simulink model "CLIK_inv_jacob_2order"  (R2021a)
settings: Solver=VariableStepAuto  StartTime=0.0  StopTime=50  RelTol=1e-3
values from neighbouring files (symbols this model uses):
  KD = kdi*eye(4)    [traiettoria.m]
  KP = kpi*eye(4)    [traiettoria.m]
  q0 = scara.ikine(T0, 'mask', [1 1 1 1 0 0])    [pseudo_traiettoria.m]    (also in traiettoria.m)
  Tc = 0.001    [pseudo_traiettoria.m]    (also in traiettoria.m)
undefined symbols (not defined in the file or in its folder): DiscIntNeverNeededParam
settings Model: Creator=Ciro  LastModifiedBy=Ciro

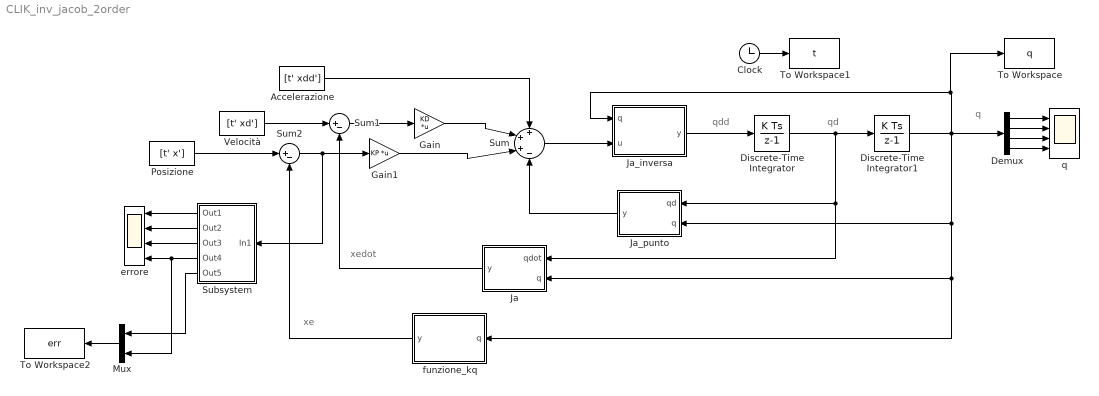
== system CLIK_inv_jacob_2order ==
  note: qd
  note: xedot
  note: qdd
  note: q
  note: xe
  Accelerazione : FromWorkspace  VariableName=[t' xdd']  SampleTime=Tc  OutputAfterFinalValue=Holding final value
  Clock : Clock
  Demux : Demux
  Discrete-Time Integrator : DiscreteIntegrator  InitialCondition=[0; 0; 0; 0]  SampleTime=Tc  ICPrevOutput=DiscIntNeverNeededParam  ICPrevScaledInput=DiscIntNeverNeededParam
  Discrete-Time Integrator1 : DiscreteIntegrator  InitialCondition=q0  SampleTime=Tc  ICPrevOutput=DiscIntNeverNeededParam  ICPrevScaledInput=DiscIntNeverNeededParam
  Gain : Gain  Gain=KD  Multiplication=Matrix(K*u)
  Gain1 : Gain  Gain=KP  Multiplication=Matrix(K*u)
  Ja : MATLAB Function  TreatAsAtomicUnit=on
  Ja_inversa : MATLAB Function  TreatAsAtomicUnit=on
  Ja_punto : MATLAB Function  TreatAsAtomicUnit=on
  Mux : Mux  Inputs=2
  Posizione : FromWorkspace  VariableName=[t' x']  SampleTime=Tc  OutputAfterFinalValue=Holding final value
  Subsystem : Subsystem
  Sum : Sum  Inputs=+++-
  Sum1 : Sum  Inputs=|+-
  Sum2 : Sum  Inputs=|+-
  To Workspace : ToWorkspace  VariableName=q  SampleTime=-1
      settings: Save2DSignal=2-D array (concatenate along first dimension)
  To Workspace1 : ToWorkspace  VariableName=t  SampleTime=-1
      settings: Save2DSignal=2-D array (concatenate along first dimension)
  To Workspace2 : ToWorkspace  VariableName=err  SampleTime=-1
      settings: Save2DSignal=2-D array (concatenate along first dimension)
  Velocità : FromWorkspace  VariableName=[t' xd']  SampleTime=Tc  OutputAfterFinalValue=Holding final value
  errore : Scope  NumInputPorts=4
  funzione_kq : MATLAB Function  TreatAsAtomicUnit=on
  q : Scope  NumInputPorts=4
  wires:
  Discrete-Time Integrator1/1 -> To Workspace/1, Ja_inversa/1(q), Demux/1, funzione_kq/1(q), Ja/2(q), Ja_punto/2(q)
  Discrete-Time Integrator/1 -> Ja/1(qdot), Ja_punto/1(qd), Discrete-Time Integrator1/1
  Ja/1(y) -> Sum1/2
  Ja_punto/1(y) -> Sum/4
  funzione_kq/1(y) -> Sum2/2
  Gain1/1 -> Sum/3
  Ja_inversa/1(y) -> Discrete-Time Integrator/1
  Sum/1 -> Ja_inversa/2(u)
  Gain/1 -> Sum/2
  Accelerazione/1 -> Sum/1
  Velocità/1 -> Sum1/1
  Demux/1 -> q/1
  Demux/2 -> q/2
  Demux/3 -> q/3
  Demux/4 -> q/4
  Sum2/1 -> Subsystem/1(In1), Gain1/1
  Sum1/1 -> Gain/1
  Posizione/1 -> Sum2/1
  Clock/1 -> To Workspace1/1
  Subsystem/3(Out3) -> errore/3
  Subsystem/2(Out2) -> errore/2
  Subsystem/1(Out1) -> errore/1
  Subsystem/4(Out4) -> Mux/2, errore/4
  Mux/1 -> To Workspace2/1
  Subsystem/5(Out5) -> Mux/1

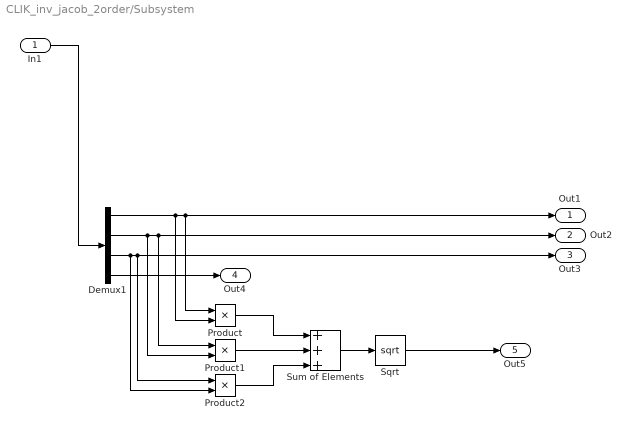
== system CLIK_inv_jacob_2order/Subsystem ==
  In1 : Inport
  Demux1 : Demux
  Product : Product
  Product1 : Product
  Product2 : Product
  Sqrt : Sqrt  SaturateOnIntegerOverflow=on
  Sum of Elements : Sum  Inputs=+++
  Out1 : Outport
  Out2 : Outport  Port=2
  Out3 : Outport  Port=3
  Out4 : Outport  Port=4
  Out5 : Outport  Port=5
  wires:
  Demux1/3 -> Product2/2, Out3/1, Product2/1
  Demux1/2 -> Product1/2, Out2/1, Product1/1
  Product/1 -> Sum of Elements/1
  Sum of Elements/1 -> Sqrt/1
  Product1/1 -> Sum of Elements/2
  Demux1/4 -> Out4/1
  Demux1/1 -> Product/2, Out1/1, Product/1
  Product2/1 -> Sum of Elements/3
  Sqrt/1 -> Out5/1
  In1/1 -> Demux1/1

== matlab function CLIK_inv_jacob_2order/Ja_inversa ==
  data: q input; u input; y output
function y = fcn(q, u)
J = [ -0.5*(sin(q(1))+sin(q(1)+q(2))) -0.5*sin(q(1)+q(2))  0  0;
       0.5*(cos(q(1))+cos(q(1)+q(2)))  0.5*cos(q(1)+q(2))  0  0;
       0                               0                  -1  0;
       1                               1                   0 -1];
y = inv(J)*u;

== matlab function CLIK_inv_jacob_2order/Ja ==
  data: qdot input; q input; y output
function y = fcn(qdot,q)
J = [ -0.5*(sin(q(1))+sin(q(1)+q(2))) -0.5*sin(q(1)+q(2))  0  0;
       0.5*(cos(q(1))+cos(q(1)+q(2)))  0.5*cos(q(1)+q(2))  0  0;
       0                               0                  -1  0;
       1                               1                   0 -1];
y = J*qdot;

== matlab function CLIK_inv_jacob_2order/Ja_punto ==
  data: qd input; q input; y output
function y = fcn(qd,q)
Jpunto = [ -0.5*(cos(q(1))*qd(1) + cos(q(1)+q(2))*(qd(1)+qd(2)))    -0.5*cos(q(1)+q(2))*(qd(1)+qd(2))  0  0;
           -0.5*(sin(q(1))*qd(1) + sin(q(1)+q(2))*(qd(1)+qd(2)))    -0.5*sin(q(1)+q(2))*(qd(1)+qd(2))  0  0;
           0                                                        0                                  0  0;
           0                                                        0                                  0  0];
y = Jpunto*qd;

== matlab function CLIK_inv_jacob_2order/funzione_kq ==
  data: q input; y output
function y = fcn(q)

xe = [0.5*(cos(q(1))+cos(q(1)+q(2)));
      0.5*(sin(q(1))+sin(q(1)+q(2)));
      0.8-q(3);
      q(1)+q(2)-q(4)];

y = xe;
